simulink model "Nov_27"  (R2022a)
settings: Solver=FixedStepAuto  StartTime=0.0  StopTime=60  FixedStep=1e-3  RelTol=1e-3  EnableMultiTasking=on
undefined symbols (not defined in the file): D0, D1, D10, D11, D12, D13, D2, D3, D4, D5, D6, D7, D8, D9, PTA0, PTA1, PTA2, PTB23, PTB9, PTC16, PTC17, PTC2, PTC3, PTC4, PTD0, PTD1, PTD2, PTD3
libraries: frdmk64flib x16, etargetslib x1
(part 1 of 3)
settings Model: ExtModeTrigDuration=5  Creator=ethan  LastModifiedBy=taimu
settings OptimizationCC: EnhancedBackFolding=on  PassReuseOutputArgsAs=Individual arguments  ZeroExternalMemoryAtStartup=off  ZeroInternalMemoryAtStartup=off  MaxStackSize=64  OptimizeBlockOrder=speed  DifferentSizesBufferReuse=on  OptimizationCustomize=off  EfficientTunableParamExpr=on
settings DebuggingCC: ParameterTunabilityLossMsg=error
settings HardwareCC: ProdBitPerPointer=32  ProdBitPerSizeT=32  ProdBitPerPtrDiffT=32  ProdLargestAtomicInteger=Long  ProdLargestAtomicFloat=Double  ProdWordSize=32  ProdHWDeviceType=ARM Compatible->ARM Cortex
settings SFSimCC: MATLABDynamicMemAlloc=off
settings RTWCC: SystemTargetFile=ert.tlc  HardwareBoard=NXP FRDM-K64F  TLCOptions="-aInlineSetEventsForThisBaseRateFcn=TLC_FALSE -aSuppressMultiTaskScheduler=TLC_FALSE  -aRateBasedStepFcn=0"  TemplateMakefile=ert_default_tmf  Toolchain=GNU Tools for ARM Embedded Processors
settings CodeAppCC: ForceParamTrailComments=on  IgnoreCustomStorageClasses=off  OperatorAnnotations=on  SimulinkDataObjDesc=on  SFDataObjDesc=on  InsertBlockDesc=on
settings ERTTargetCC: ExtModeTransport=4  ExtModeMexFile=sendToCommService

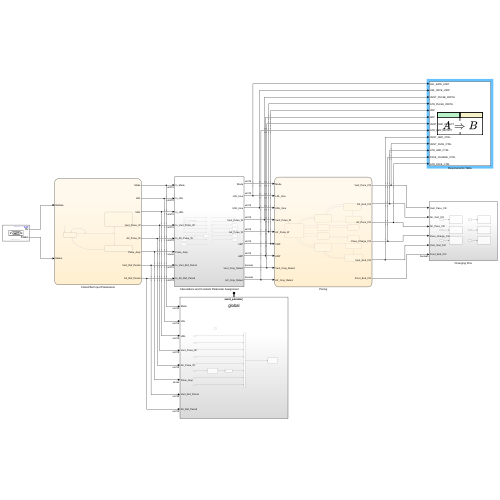
[thumbnail: Simulink's stored preview of the top-level diagram]
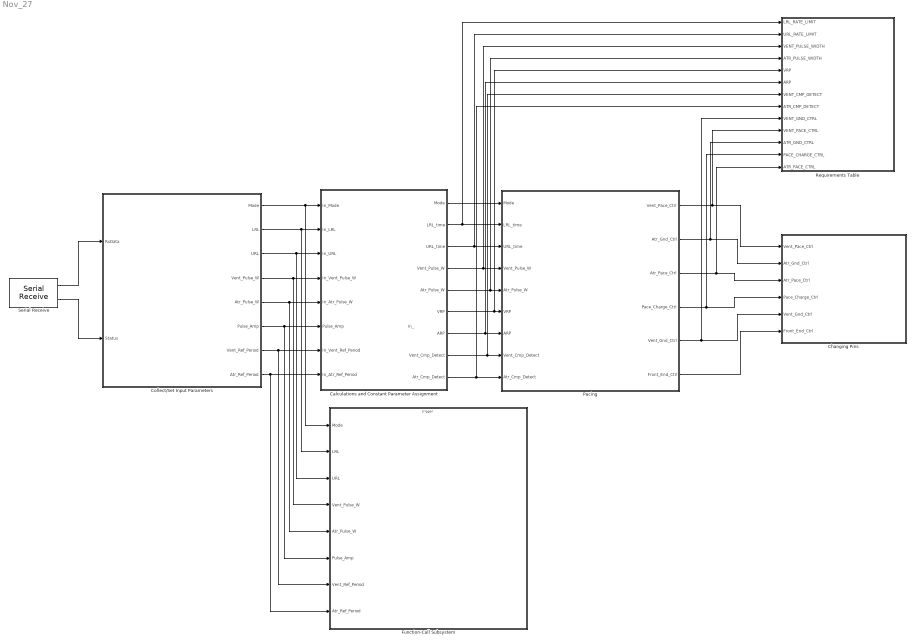
== system Nov_27 ==
  note: In_
  Calculations and Constant Parameter Assignment : Subsystem
  Changing Pins : Subsystem
  Collect/Set Input Parameters : Stateflow chart  TreatAsAtomicUnit=on
      settings: PortSchema="{\"entries\":[{\"content\":{\"sides\":[{\"content\":{\"connectorIds\":[\"In1\",\"In2\"]},\"type\":\"ConnectorPlacement.EquallySpacedRectSide\",\"uuid\":\"dc51e4f5-5341-418f-80a9-38d3dc8e9b6e\"},{\"content\":{\"connectorIds\":[\"Out1\",\"Out8\",\"Out4\",\"Out6\",\"Out2\",\"Out5\",\"Out7\",\"Out3\"],\"side\":\"RIGHT\"},\"type\":\"ConnectorPlacement.EquallySpacedRectSide\",\"uuid\":\"313c6298-b0b7-4ff0-85ba-dbaa1c18177a\"},{\"content\":{\"connectorIds\":[],\"side\":\"TOP\"},\"type\":\"ConnectorPlacement.EquallySpacedRectSide\",\"uuid\":\"6f377806-6de9-4b84-8111-50855010f7f2\"}]},\"type\":\"ConnectorPlacement.EquallySpacedConnector\",\"uuid\":\"8b0403f6-9322-46f9-82a4-778a28822a3d\"}],\"packageUris\":[\"http://schema.mathworks.com/mf0/Connector/R2020b\"],\"version\":\"1.0\"}"
  Function-Call Subsystem : Subsystem  TreatAsAtomicUnit=on
  Pacing : Stateflow chart  TreatAsAtomicUnit=on
      settings: PortSchema="{\"entries\":[{\"content\":{\"sides\":[{\"content\":{\"connectorIds\":[\"In1\",\"In4\",\"In5\",\"In3\",\"In2\",\"In7\",\"In6\",\"In8\",\"In9\"]},\"type\":\"ConnectorPlacement.EquallySpacedRectSide\",\"uuid\":\"cbd26b3d-27cb-4744-9a6d-2e29f16e2c2e\"},{\"content\":{\"connectorIds\":[\"Out1\",\"Out2\",\"Out3\",\"Out4\",\"Out5\",\"Out6\"],\"side\":\"RIGHT\"},\"type\":\"ConnectorPlacement.EquallySpacedRectSide\",\"uuid\":\"25c89074-e17e-4898-a31a-c42a3e343a2e\"},{\"content\":{\"connectorIds\":[],\"side\":\"TOP\"},\"type\":\"ConnectorPlacement.EquallySpacedRectSide\",\"uuid\":\"e4014b57-3770-4bf4-bd9b-5c9114757f0a\"}]},\"type\":\"ConnectorPlacement.EquallySpacedConnector\",\"uuid\":\"9ef350bf-8d26-4971-b7d1-0d0774d6b5a5\"}],\"packageUris\":[\"http://schema.mathworks.com/mf0/Connector/R2020b\"],\"version\":\"1.0\"}"
  Requirements Table : Requirements Table  TreatAsAtomicUnit=on
  Serial Receive : frdmk64flib/Serial Receive  SCIModule=0  Baudrate=uint32(9600)  Parity=None  StopBits=1  HardwareFlowControl=None  ByteOrder=LittleEndian  DataType=uint8  DataLength=20  BlockingMode=off  OutputStatus=on  SampleTime=-1
  wires:
  Serial Receive/1 -> Collect/Set Input Parameters/1(RxData)
  Serial Receive/2 -> Collect/Set Input Parameters/2(Status)
  Pacing/1(Vent_Pace_Ctrl) -> Requirements Table/10(VENT_PACE_CTRL), Changing Pins/1(Vent_Pace_Ctrl)
  Pacing/2(Atr_Gnd_Ctrl) -> Requirements Table/11(ATR_GND_CTRL), Changing Pins/2(Atr_Gnd_Ctrl)
  Pacing/3(Atr_Pace_Ctrl) -> Requirements Table/13(ATR_PACE_CTRL), Changing Pins/3(Atr_Pace_Ctrl)
  Pacing/4(Pace_Charge_Ctrl) -> Requirements Table/12(PACE_CHARGE_CTRL), Changing Pins/4(Pace_Charge_Ctrl)
  Pacing/5(Vent_Gnd_Ctrl) -> Requirements Table/9(VENT_GND_CTRL), Changing Pins/5(Vent_Gnd_Ctrl)
  Pacing/6(Front_End_Ctrl) -> Changing Pins/6(Front_End_Ctrl)
  Collect/Set Input Parameters/1(Mode) -> Function-Call Subsystem/1(Mode), Calculations and Constant Parameter Assignment/1(In_Mode)
  Collect/Set Input Parameters/5(Pulse_Amp) -> Function-Call Subsystem/6(Pulse_Amp), Calculations and Constant Parameter Assignment/6(Pulse_Amp)
  Collect/Set Input Parameters/2(Atr_Pulse_W) -> Function-Call Subsystem/5(Atr_Pulse_W), Calculations and Constant Parameter Assignment/5(In_Atr_Pulse_W)
  Collect/Set Input Parameters/6(Vent_Pulse_W) -> Function-Call Subsystem/4(Vent_Pulse_W), Calculations and Constant Parameter Assignment/4(In_Vent_Pulse_W)
  Collect/Set Input Parameters/8(LRL) -> Function-Call Subsystem/2(LRL), Calculations and Constant Parameter Assignment/2(In_LRL)
  Collect/Set Input Parameters/4(URL) -> Function-Call Subsystem/3(URL), Calculations and Constant Parameter Assignment/3(In_URL)
  Collect/Set Input Parameters/3(Atr_Ref_Period) -> Function-Call Subsystem/8(Atr_Ref_Period), Calculations and Constant Parameter Assignment/8(In_Atr_Ref_Period)
  Collect/Set Input Parameters/7(Vent_Ref_Period) -> Function-Call Subsystem/7(Vent_Ref_Period), Calculations and Constant Parameter Assignment/7(In_Vent_Ref_Period)
  Calculations and Constant Parameter Assignment/1(Mode) -> Pacing/1(Mode)
  Calculations and Constant Parameter Assignment/2(LRL_time) -> Requirements Table/1(LRL_RATE_LIMIT), Pacing/4(LRL_time)
  Calculations and Constant Parameter Assignment/3(URL_time) -> Requirements Table/2(URL_RATE_LIMIT), Pacing/5(URL_time)
  Calculations and Constant Parameter Assignment/4(Vent_Pulse_W) -> Requirements Table/3(VENT_PULSE_WIDTH), Pacing/3(Vent_Pulse_W)
  Calculations and Constant Parameter Assignment/5(Atr_Pulse_W) -> Requirements Table/4(ATR_PULSE_WIDTH), Pacing/2(Atr_Pulse_W)
  Calculations and Constant Parameter Assignment/6(VRP) -> Requirements Table/5(VRP), Pacing/7(VRP)
  Calculations and Constant Parameter Assignment/7(ARP) -> Requirements Table/6(ARP), Pacing/6(ARP)
  Calculations and Constant Parameter Assignment/8(Vent_Cmp_Detect) -> Requirements Table/7(VENT_CMP_DETECT), Pacing/8(Vent_Cmp_Detect)
  Calculations and Constant Parameter Assignment/9(Atr_Cmp_Detect) -> Requirements Table/8(ATR_CMP_DETECT), Pacing/9(Atr_Cmp_Detect)

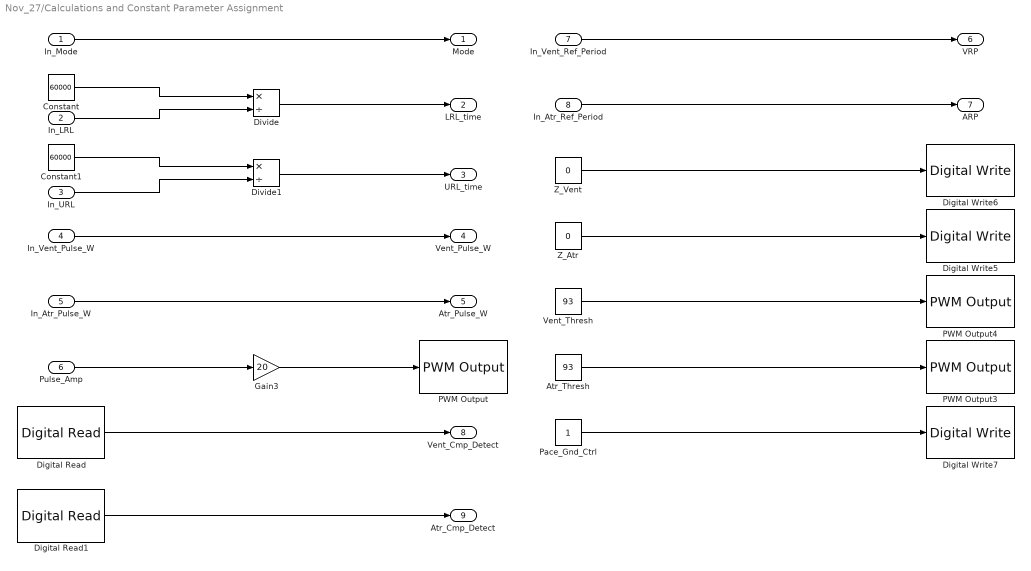
== system Nov_27/Calculations and Constant Parameter Assignment ==
  In_Mode : Inport  OutDataTypeStr=uint16
  In_LRL : Inport  Port=2  OutDataTypeStr=uint16
  In_URL : Inport  Port=3  OutDataTypeStr=uint16
  In_Vent_Pulse_W : Inport  Port=4  OutDataTypeStr=uint16  LockScale=on
  In_Atr_Pulse_W : Inport  Port=5  OutDataTypeStr=uint16
  Pulse_Amp : Inport  Port=6  OutDataTypeStr=single
  In_Vent_Ref_Period : Inport  Port=7  OutDataTypeStr=uint16
  In_Atr_Ref_Period : Inport  Port=8  OutDataTypeStr=uint16
  Atr_Thresh : Constant  Value=93
  Constant : Constant  Value=60000  OutDataTypeStr=uint16
  Constant1 : Constant  Value=60000  OutDataTypeStr=uint16
  Digital Read : frdmk64flib/Digital Read  Whichpin=PTC17 (D1)  SampleTime=-1
  Digital Read1 : frdmk64flib/Digital Read  Whichpin=PTC16 (D0)  SampleTime=-1
  Digital Write5 : frdmk64flib/Digital Write  Whichpin=PTB23 (D4)
  Digital Write6 : frdmk64flib/Digital Write  Whichpin=PTC3 (D7)
  Digital Write7 : frdmk64flib/Digital Write  Whichpin=PTD0 (D10)
  Divide : Product  Inputs=*/  OutDataTypeStr=uint16
  Divide1 : Product  Inputs=*/  OutDataTypeStr=uint16
  Gain3 : Gain  Gain=20
  PWM Output : frdmk64flib/PWM Output  Whichpin=PTA2 (D5)  InitialFrequency=2000  InitialDutyCycle=0
  PWM Output3 : frdmk64flib/PWM Output  Whichpin=PTC2 (D6)  InitialFrequency=2000  InitialDutyCycle=0
  PWM Output4 : frdmk64flib/PWM Output  Whichpin=PTA1 (D3)  InitialFrequency=2000  InitialDutyCycle=0
  Pace_Gnd_Ctrl : Constant
  Vent_Thresh : Constant  Value=93
  Z_Atr : Constant  Value=0
  Z_Vent : Constant  Value=0
  Mode : Outport  OutDataTypeStr=uint16
  LRL_time : Outport  Port=2  OutDataTypeStr=uint16
  URL_time : Outport  Port=3  OutDataTypeStr=uint16
  Vent_Pulse_W : Outport  Port=4  OutDataTypeStr=uint16
  Atr_Pulse_W : Outport  Port=5  OutDataTypeStr=uint16
  VRP : Outport  Port=6  OutDataTypeStr=uint16
  ARP : Outport  Port=7  OutDataTypeStr=uint16
  Vent_Cmp_Detect : Outport  Port=8  OutDataTypeStr=boolean
  Atr_Cmp_Detect : Outport  Port=9  OutDataTypeStr=boolean
  wires:
  In_Mode/1 -> Mode/1
  Pulse_Amp/1 -> Gain3/1
  In_Atr_Pulse_W/1 -> Atr_Pulse_W/1
  In_Vent_Pulse_W/1 -> Vent_Pulse_W/1
  In_Vent_Ref_Period/1 -> VRP/1
  In_Atr_Ref_Period/1 -> ARP/1
  Gain3/1 -> PWM Output/1
  Digital Read/1 -> Vent_Cmp_Detect/1
  Z_Atr/1 -> Digital Write5/1
  Z_Vent/1 -> Digital Write6/1
  Vent_Thresh/1 -> PWM Output4/1
  Pace_Gnd_Ctrl/1 -> Digital Write7/1
  Atr_Thresh/1 -> PWM Output3/1
  Constant/1 -> Divide/1
  In_LRL/1 -> Divide/2
  Divide/1 -> LRL_time/1
  Constant1/1 -> Divide1/1
  Divide1/1 -> URL_time/1
  In_URL/1 -> Divide1/2
  Digital Read1/1 -> Atr_Cmp_Detect/1

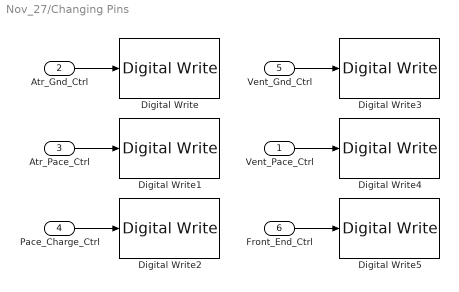
== system Nov_27/Changing Pins ==
  Vent_Pace_Ctrl : Inport
  Atr_Gnd_Ctrl : Inport  Port=2
  Atr_Pace_Ctrl : Inport  Port=3
  Pace_Charge_Ctrl : Inport  Port=4
  Vent_Gnd_Ctrl : Inport  Port=5
  Front_End_Ctrl : Inport  Port=6  OutDataTypeStr=boolean
  Digital Write : frdmk64flib/Digital Write  Whichpin=PTD2 (D11)
  Digital Write1 : frdmk64flib/Digital Write  Whichpin=PTA0 (D8)
  Digital Write2 : frdmk64flib/Digital Write  Whichpin=PTB9 (D2)
  Digital Write3 : frdmk64flib/Digital Write  Whichpin=PTD3 (D12)
  Digital Write4 : frdmk64flib/Digital Write  Whichpin=PTC4 (D9)
  Digital Write5 : frdmk64flib/Digital Write  Whichpin=PTD1 (D13)
  wires:
  Atr_Gnd_Ctrl/1 -> Digital Write/1
  Atr_Pace_Ctrl/1 -> Digital Write1/1
  Pace_Charge_Ctrl/1 -> Digital Write2/1
  Vent_Gnd_Ctrl/1 -> Digital Write3/1
  Vent_Pace_Ctrl/1 -> Digital Write4/1
  Front_End_Ctrl/1 -> Digital Write5/1

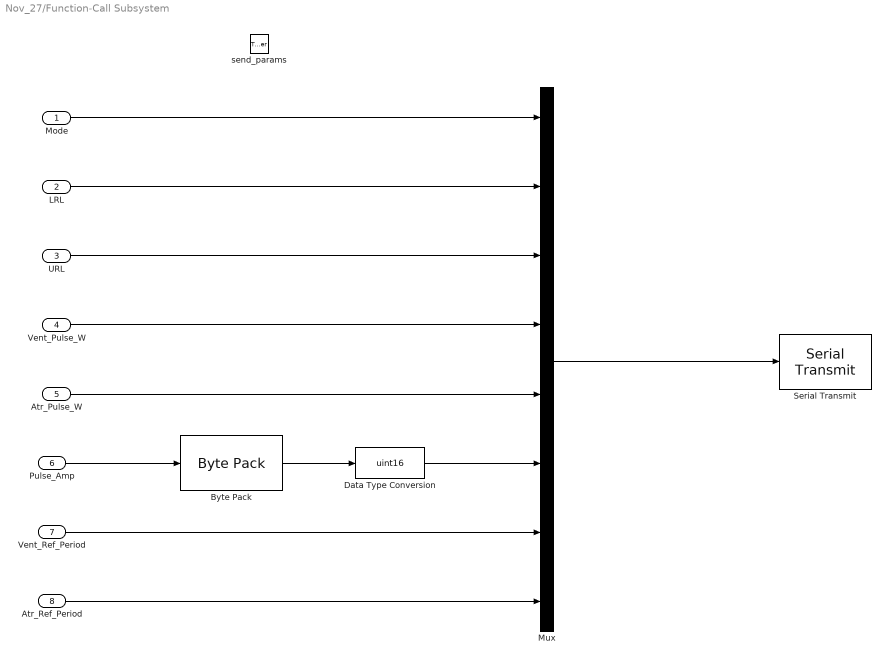
== system Nov_27/Function-Call Subsystem ==
  Mode : Inport  OutDataTypeStr=uint16
  LRL : Inport  Port=2  OutDataTypeStr=uint16
  URL : Inport  Port=3  OutDataTypeStr=uint16
  Vent_Pulse_W : Inport  Port=4  OutDataTypeStr=uint16  LockScale=on
  Atr_Pulse_W : Inport  Port=5  OutDataTypeStr=uint16
  Pulse_Amp : Inport  Port=6  OutDataTypeStr=single
  Vent_Ref_Period : Inport  Port=7  OutDataTypeStr=uint16
  Atr_Ref_Period : Inport  Port=8  OutDataTypeStr=uint16
  send_params : TriggerPort  TriggerType=function-call  IsSimulinkFunction=on  FunctionName=send_params  VariantControl=(inherit)
  Byte Pack : etargetslib/Byte Pack  datatypes={'single'}  byteAlign=1
  Data Type Conversion : DataTypeConversion  OutDataTypeStr=uint16  SaturateOnIntegerOverflow=off  RndMeth=Floor
  Mux : Mux  Inputs=8
  Serial Transmit : frdmk64flib/Serial Transmit  SCIModule=0  Baudrate=uint32(9600)  Parity=None  StopBits=1  HardwareFlowControl=None  ByteOrder=LittleEndian  BlockingMode=on  OutputStatus=off
  wires:
  Byte Pack/1 -> Data Type Conversion/1
  Data Type Conversion/1 -> Mux/6
  LRL/1 -> Mux/2
  Mux/1 -> Serial Transmit/1
  URL/1 -> Mux/3
  Mode/1 -> Mux/1
  Atr_Pulse_W/1 -> Mux/5
  Pulse_Amp/1 -> Byte Pack/1
  Atr_Ref_Period/1 -> Mux/8
  Vent_Pulse_W/1 -> Mux/4
  Vent_Ref_Period/1 -> Mux/7
